simulink library "Source_Lib"  (R2020b)
settings: Solver=VariableStepAuto  StartTime=0.0  StopTime=10.0  RelTol=1e-3
values from neighbouring files (symbols this model uses):
  fb = fn    [Init_Base_SM.m]
  Ib2 = Sb / (3*Vb2)    [Init_Base_SM.m]
undefined symbols (not defined in the file or in its folder): Cmu0, delta0, GOV1_K2, ia0, ib0, ic0, pha0, phb0, phc0, Theta0_deg, Time_Step, V0_pu, Vfu0
libraries: powerlib x41, Control_Lib x14, spsPower3phInstantaneousLib x3, spsSynchronousMachinepuFundamentalLib x2
(part 1 of 2)
settings Model: Creator=abruyere  LastModifiedBy=Frederic_Colas
settings DebuggingCC: ArithmeticOperatorsInVariantConditions=warning
settings SFSimCC: CustomCodeUndefinedFunction=UseInterfaceOnly

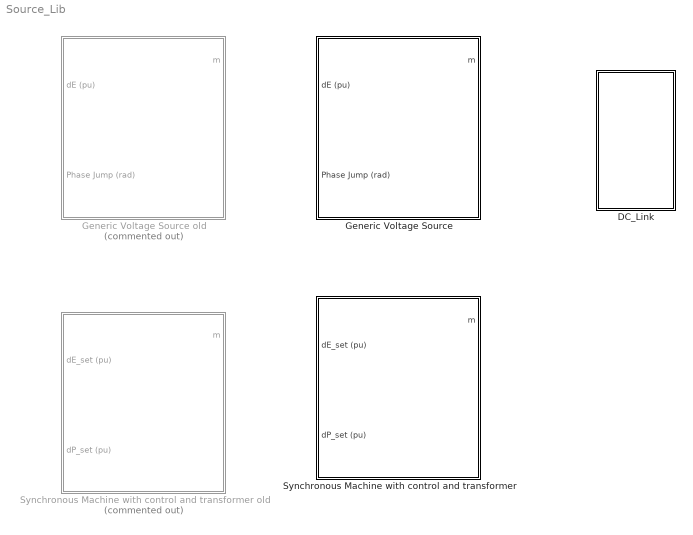
== system Source_Lib ==
  DC_Link : Subsystem  mask{Udc=640e3, Pb=1e6, H_DC=30}
      mask prompts: Udc "Nominal Voltage (V)"; Pb "Nominal Power (W)"; H_DC "DC inertia (ms)"
      mask init:
      | if (H_DC == 0)
      |     set_param([gcb '/C_1'],'Commented','on');
      |     set_param([gcb '/C_2'],'Commented','on');
      |     set_param([gcb '/Udc_1'],'Commented','on');
      |     set_param([gcb '/Udc_2'],'Commented','on');
      | elseif (H_DC == inf)
      |     set_param([gcb '/C_1'],'Commented','on');
      |     set_param([gcb '/C_2'],'Commented','on');
      |     set_param([gcb '/Udc_1'],'Commented','off');
      |     set_param([gcb '/Udc_2'],'Commented','off');
      | else
      |    C_DC = H_DC/1000*Pb/(1/2*Udc^2);
      |    set_param([gcb '/C_1'],'Commented','off','Capacitance',num2str(C_DC*2));
      |    set_param([gcb '/C_2'],'Commented','off','Capacitance',num2str(C_DC*2));
      |    set_param([gcb '/Udc_1'],'Commented','on');
      |    set_param([gcb '/Udc_2'],'Commented','on');
      | end
  Generic Voltage Source : Subsystem  mask(GenericVoltageSource){SourceNature_str=INFINITE, fn=50, Sn=1e9, Un=400e3, H_s=5, DroopOnOff=on, R_percent=4, TN=1, TD=2, Time_Step=50e-6, LFpopup=Swing, P0=0, Q0=0, V0=1, Theta0=0}
      mask prompts: SourceNature_str "Nature of the voltage source"; fn "Nominal frequency fn [Hz]"; Sn "Nominal apparent power Sn [VA]"; Un "Nominal voltage Un [V RMS Ph2Ph]"; H_s "Inertia H [s]"; DroopOnOff "Frequency DROOP activation"; R_percent "Droop gain Kp [%]"; TN "Network time constant Lead [s]"; TD "Network time constant Lag [s]"; Time_Step "Output Delay (s)"; P0 "Active power P0 (pu)"; Q0 "Reactive power Q0 (pu)"; V0 "Initial Voltage (pu)"; Theta0 "Initial angle (°)"
      mask init:
      | % Update Name of LF bus for internal purpose
      | NameStr = [get_param(gcb,'Name')];% '_LF'];
      | set_param([gcb '/Load Flow Bus'],'ID',NameStr);  
      | 
      | % Base specification
      | fb = fn;                % [Hz] base frequency
      | Sb = Sn;                % [VA] base power
      | Ub = Un;                % [V] base ph2ph voltage
      | Vb = Un/sqrt(3);        % [V] base ph2N voltage
      | Ib = Sb/(3*Vb);         % [A] base current
      | Zb = Vb*Ib;             % [Ohm] base impedance
      | 
      | % Set the frequency droop gain
      | R = R_percent / 100;
      | 
      | %Initialize correctly the LoadFlow bus parameters connected to PCC
      |     VLF = V0;
      |     ThetaLF = Theta0;
      |     if (LFpopup == 'PQ')
      |         VLF = 1;
      |         ThetaLF = 0;
      |     elseif (LFpopup == 'PV')
      |         VLF = V0;
      |         ThetaLF = 0;        
      |     end
      |     set_param([gcb '/Load Flow Bus'],'Vref',num2str(VLF),'Vangle',num2str(ThetaLF));
      | 
      | 
      | % Update mask display:
      | % mo = get_param(gcb,'MaskObject');
      | % Generate string to display LF results on Mask
      |     mo = get_param(gcb,'MaskObject');
      |     mo.getDialogControl('LF_pcc_str').Prompt = ['V0 = ', num2str(V0),' pu, Angle = ', num2str(Theta0),'°'];
      |     mo.getDialogControl('LF_pcc_Power_str').Prompt = ['P0 = ', num2str(P0),' pu, Q0 = ', num2str(Q0),' pu'];
      mask TypeOptions SourceNature_str: INFINITE | INERTIAL
      mask Callback SourceNature_str:
      | % Get the mask parameter values. This is a cell
      | %   array of character vectors.
      | maskStr = get_param(gcb,'SourceNature_str');
      | p=Simulink.Mask.get(gcb);
      | 
      | % The pop-up menu is the first mask parameter.
      | %   Check the value selected in the pop-up
      | if strcmp(maskStr,'INFINITE')
      |     p.getDialogControl('Inertial').Visible='off';
      |    %p.getParameter('H_s').Visible='off';
      |    %p.getParameter('DroopOnOff').Visible='off';
      |    %DroopOnOff = 'off';
      |    %p.getParameter('R_percent').Visible='off';
      |    %p.getParameter('TN').Visible='off';
      |    %p.getParameter('TD').Visible='off';
      |    set_param([gcb '/SourceNature'],'Value','1')
      | else
      |    %p.getParameter('H_s').Visible='on';
      |    %p.getParameter('DroopOnOff').Visible='on';
      |    %DroopOnOff = 'on';
      |    %p.getParameter('R_percent').Visible='on';
      |    %p.getParameter('TN').Visible='on';
      |    %p.getParameter('TD').Visible='on';
      |    p.getDialogControl('Inertial').Visible='on';
      |    set_param([gcb '/SourceNature'],'Value','2')
      | end
      mask Callback DroopOnOff:
      | % Get the mask parameter values. This is a cell
      | %   array of character vectors.
      | maskStr = get_param(gcb,'DroopOnOff');
      | p=Simulink.Mask.get(gcb);
      | 
      | if strcmp(maskStr,'on'),
      |     p.getParameter('R_percent').Enabled='on';
      | else
      |     p.getParameter('R_percent').Enabled='off';
      | end
      mask TypeOptions LFpopup: Swing | PQ | PV
      mask Callback LFpopup:
      | % Get the mask parameter values. This is a cell
      | %   array of character vectors.
      | maskStr = get_param(gcb,'LFpopup');
      | p=Simulink.Mask.get(gcb);
      | 
      | % The pop-up menu is the first mask parameter.
      | %   Check the value selected in the pop-up
      | if strcmp(maskStr,'Swing'),
      | 
      |     % Set the visibility of both parameters on when
      |     %   User-defined is selected in the pop-up.
      |     p.getParameter('P0').Visible='off';
      |     p.getParameter('Q0').Visible='off';
      |     p.getParameter('V0').Visible='on';
      |     p.getParameter('Theta0').Visible='on';
      |     set_param([gcb '/Source_For_LF'],'BusType','swing');
      | 
      | elseif strcmp(maskStr,'PQ'),
      | 
      |     % Set the visibility of both parameters on when
      |     %   User-defined is selected in the pop-up.
      |     p.getParameter('P0').Visible='on';
      |     p.getParameter('Q0').Visible='on';
      |     p.getParameter('V0').Visible='off';
      |     p.getParameter('Theta0').Visible='off';
      |     set_param([gcb '/Source_For_LF'],'BusType','PQ');
      | 
      |     % Turn off the visibility of the Value field
      |     %   when User-defined is not selected.
      | else
      | 
      |     % Set the visibility of both parameters on when
      |     %   User-defined is selected in the pop-up.
      |     p.getParameter('P0').Visible='on';
      |     p.getParameter('Q0').Visible='off';
      |     p.getParameter('V0').Visible='on';
      |     p.getParameter('Theta0').Visible='off';
      |     set_param([gcb '/Source_For_LF'],'BusType','PV');
      | 
      | end
      mask DialogControl Container8 Prompt: Nominal Value
      mask DialogControl Inertial Prompt: Inertial source parameters
      mask DialogControl LF_Param Prompt: Loadflow
      mask DialogControl Control1 Prompt: Initial Operating Point
      mask DialogControl Container6 Prompt: PCC
      mask DialogControl LF_pcc_str Prompt: V0 = 1 pu, Angle = 0°
      mask DialogControl LF_pcc_Power_str Prompt: P0 = 0 pu, Q0 = 0 pu
      mask DialogControl Control4 Prompt: Update Loadflow
      mask DialogControl Control4 Callback: LoadFlow_VSC
      mask Display:
      | if (SourceNature_str == 1)
      |     image(imread('infinite.png'));
      |     color('blue')
      |     text(0.3,0.10,'Infinite bus')
      | else
      |     image(imread('inertia.png'));
      |     color('blue')
      |     text(0.3,0.10,'Inertia Emulation')
      | end
      | 
      | port_label('input',1,'\DeltaE (pu)','texmode','on');
      | port_label('input',2,'\Delta\theta (rad)','texmode','on');
      | port_label('output',1,'m');
      | port_label('rconn',1,'A');
      | port_label('rconn',2,'B');
      | port_label('rconn',3,'C');
  Generic Voltage Source old : Subsystem  Commented=on  mask(GenericVoltageSource){SourceNature_str=INFINITE, fn=50, Sn=1e9, Un=400e3, Time_Step=Time_Step, H_s=5, DroopOnOff=on, R_percent=4, TN=1, TD=2, LFpopup=Swing, P0=-491545376.7896, Q0=82825649.5509, V0=1, Theta0=0}
      mask prompts: SourceNature_str "Nature of the voltage source"; fn "Nominal frequency fn [Hz]"; Sn "Nominal apparent power Sn [VA]"; Un "Nominal voltage Un [V RMS Ph2Ph]"; Time_Step "Sample Time (s)"; H_s "Inertia H [s]"; DroopOnOff "Frequency DROOP activation"; R_percent "Droop gain Kp [%]"; TN "Network time constant Lead [s]"; TD "Network time constant Lag [s]"; P0 "Active power P0 (pu)"; Q0 "Reactive power Q0 (pu)"; V0 "Initial Voltage (pu)"; Theta0 "Initial angle (°)"
      mask init:
      | % Update Name of LF bus for internal purpose
      | NameStr = [get_param(gcb,'Name')];% '_LF'];
      | set_param([gcb '/Load Flow Bus'],'ID',NameStr);  
      | 
      | % Base specification
      | fb = fn;                % [Hz] base frequency
      | Sb = Sn;                % [VA] base power
      | Ub = Un;                % [V] base ph2ph voltage
      | Vb = Un/sqrt(3);        % [V] base ph2N voltage
      | Ib = Sb/(3*Vb);         % [A] base current
      | Zb = Vb*Ib;             % [Ohm] base impedance
      | 
      | % Set the frequency droop gain
      | R = R_percent / 100;
      | 
      | %Initialize correctly the LoadFlow bus parameters connected to PCC
      |     VLF = V0_pu;
      |     ThetaLF = Theta0_deg;
      |     if (LFpopup == 'PQ')
      |         VLF = 1;
      |         ThetaLF = 0;
      |     elseif (LFpopup == 'PV')
      |         VLF = V0_pu;
      |         ThetaLF = 0;        
      |     end
      |     set_param([gcb '/Load Flow Bus'],'Vref',num2str(VLF),'Vangle',num2str(ThetaLF));
      | 
      | 
      | % Update mask display:
      | % mo = get_param(gcb,'MaskObject');
      mask TypeOptions SourceNature_str: INFINITE | INERTIAL
      mask Callback SourceNature_str:
      | % Get the mask parameter values. This is a cell
      | %   array of character vectors.
      | maskStr = get_param(gcb,'SourceNature_str');
      | p=Simulink.Mask.get(gcb);
      | 
      | % The pop-up menu is the first mask parameter.
      | %   Check the value selected in the pop-up
      | if strcmp(maskStr,'INFINITE')
      |     p.getDialogControl('Inertial').Visible='off';
      |    %p.getParameter('H_s').Visible='off';
      |    %p.getParameter('DroopOnOff').Visible='off';
      |    %DroopOnOff = 'off';
      |    %p.getParameter('R_percent').Visible='off';
      |    %p.getParameter('TN').Visible='off';
      |    %p.getParameter('TD').Visible='off';
      |    set_param([gcb '/SourceNature'],'Value','1')
      | else
      |    %p.getParameter('H_s').Visible='on';
      |    %p.getParameter('DroopOnOff').Visible='on';
      |    %DroopOnOff = 'on';
      |    %p.getParameter('R_percent').Visible='on';
      |    %p.getParameter('TN').Visible='on';
      |    %p.getParameter('TD').Visible='on';
      |    p.getDialogControl('Inertial').Visible='on';
      |    set_param([gcb '/SourceNature'],'Value','2')
      | end
      mask Callback DroopOnOff:
      | % Get the mask parameter values. This is a cell
      | %   array of character vectors.
      | maskStr = get_param(gcb,'DroopOnOff');
      | p=Simulink.Mask.get(gcb);
      | 
      | if strcmp(maskStr,'on'),
      |     p.getParameter('R_percent').Enabled='on';
      | else
      |     p.getParameter('R_percent').Enabled='off';
      | end
      mask TypeOptions LFpopup: Swing | PQ | PV
      mask Callback LFpopup:
      | % Get the mask parameter values. This is a cell
      | %   array of character vectors.
      | maskStr = get_param(gcb,'LFpopup');
      | p=Simulink.Mask.get(gcb);
      | 
      | % The pop-up menu is the first mask parameter.
      | %   Check the value selected in the pop-up
      | if strcmp(maskStr,'Swing'),
      | 
      |     % Set the visibility of both parameters on when
      |     %   User-defined is selected in the pop-up.
      |     p.getParameter('P0').Visible='off';
      |     p.getParameter('Q0').Visible='off';
      |     p.getParameter('V0').Visible='on';
      |     p.getParameter('Theta0').Visible='on';
      |     set_param([gcb '/Source_For_LF'],'BusType','swing');
      | 
      | elseif strcmp(maskStr,'PQ'),
      | 
      |     % Set the visibility of both parameters on when
      |     %   User-defined is selected in the pop-up.
      |     p.getParameter('P0').Visible='on';
      |     p.getParameter('Q0').Visible='on';
      |     p.getParameter('V0').Visible='off';
      |     p.getParameter('Theta0').Visible='off';
      |     set_param([gcb '/Source_For_LF'],'BusType','PQ');
      | 
      |     % Turn off the visibility of the Value field
      |     %   when User-defined is not selected.
      | else
      | 
      |     % Set the visibility of both parameters on when
      |     %   User-defined is selected in the pop-up.
      |     p.getParameter('P0').Visible='on';
      |     p.getParameter('Q0').Visible='off';
      |     p.getParameter('V0').Visible='on';
      |     p.getParameter('Theta0').Visible='off';
      |     set_param([gcb '/Source_For_LF'],'BusType','PV');
      | 
      | end
      mask DialogControl Container8 Prompt: Nominal Value
      mask DialogControl Inertial Prompt: Inertial source parameters
      mask DialogControl LF_Param Prompt: Loadflow
      mask Display:
      | if (SourceNature_str == 1)
      |     image(imread('infinite.png'));
      |     color('blue')
      |     text(0.3,0.10,'Infinite bus')
      | else
      |     image(imread('inertia.png'));
      |     color('blue')
      |     text(0.3,0.10,'Inertia Emulation')
      | end
      | 
      | port_label('input',1,'\DeltaE (pu)','texmode','on');
      | port_label('input',2,'\Delta\theta (rad)','texmode','on');
      | port_label('output',1,'m');
      | port_label('rconn',1,'A');
      | port_label('rconn',2,'B');
      | port_label('rconn',3,'C');
  Synchronous Machine with control and transformer : Subsystem  mask(SM){Sn=900e6, Pn=900e6, fn=50, SM_Unom=20e3, Paux=0.01, SM_Rs=0.0025, SM_Ll=0.2, SM_Lmd=1.6, SM_Lmq=1.5, SM_Rf=0.006, SM_Llfd=0.1067, SM_Rkd=0.0177, SM_Llkd=0.1, SM_Rkq1=0.013, SM_Llkq1=0.4565, SM_Rkq2=0.0217, SM_Llkq2=0.0583, SM_H=6.5, SM_F=0, SM_p=1, Un1=20e3, Un2=400e3, Rt_pu=0, Lt_pu=0.15, Lm_pu=500, Rm_pu=500, GOV_Kpf=-25, GOV_tau1=0.1, GOV_tau3=0.2, GOV_tau4=0.05, GOV_K2=0.7, GOV_tau5=7, GOV_K3=0.4, GOV_tau6=0.4, ST1_Ka=200, ST1_taur=0.01, OP_Vfu=0, PSS_K=20, PSS_tau1=0.05, PSS_tau2=0.02, PSS_tau3=3, PSS_tau4=5.4, PSS_tau5=0.05, PSS_tau6=0.01, LFpopup=PV, P0=0.9, Q0=-0.064025, V0=1, Theta0=3.6743}
      mask prompts: Sn "Nominal apparent power (VA)"; Pn "Nominal active power (W)"; fn "Frequency (Hz)"; SM_Unom "Line-to-line voltage (Vrms)"; Paux "Auxilary charge  (p.u)"; SM_Rs "Stator resistance : Rs(pu)"; SM_Ll "Stator leakage inductance : Ll(pu)"; SM_Lmd "Magnetic inductance in d-axis  : Lmd(pu)"; SM_Lmq "Magnetic inductance in q-axis  : Lmq(pu)"; SM_Rf "Field resistance : Rf(pu)"; SM_Llfd "Field leakage inductance  : Llfd(pu)"; SM_Rkd "d-axis damper resistance : Rkd(pu)"; SM_Llkd "d-axis damper leakage inductance : Llkd(pu)"; SM_Rkq1 "1st q-axis damper resistance:  Rkq1(pu)"; SM_Llkq1 "1st q-axis damper leakage inductance : Lkq1(pu)"; SM_Rkq2 "2nd  q-axis damper resistance :  Rkq2(pu)"; SM_Llkq2 "2nd q-axis damper leakage inductance :  Llkq2(pu)"; SM_H "Inertia coefficient : H(s)"; SM_F "Friction  factor : F(pu)"; SM_p "Poles pairs : p()"; Un1 "Primary line-to-line voltage (Vrms)"; Un2 "Secondary line-to-line voltage (Vrms)"; Rt_pu "Resistance : R(pu)"; Lt_pu "Leakage inductance : L(pu)"; Lm_pu "Magnetization resistance : Rm(pu)"; Rm_pu "Magnetization resistance : Lm(pu)"; GOV_Kpf "Power frecuency characteristic : Kpf"; GOV_tau1 "Lag time constant : tau1(s)"; GOV_tau3 "Lag time constant : tau3(s)"; GOV_tau4 "Steam flow time constant : tau4(s)"; GOV_K2 "Intermediary Pressure Reheater power fraction : K2"; GOV_tau5 "Intermediary Pressure Reheater time constant : tau5(s)"; GOV_K3 "Low Pressure Reheater power fraction : K3"; GOV_tau6 "Intermediary Pressure Reheater time constant : tau6(s)"; ST1_Ka "Main regulator gain : Ka"; ST1_taur "Filter time constant : taur(s)"; PSS_K "Gain"; PSS_tau1 "tau1"; PSS_tau2 "tau2"; PSS_tau3 "tau3"; PSS_tau4 "tau4"; PSS_tau5 "tau5"; PSS_tau6 "tau6"; P0 "Initial Active Power (pu)"; Q0 "Initial Reactive Power (pu)"; V0 "Initial Voltage (pu)"; Theta0 "Initial Angle (°)"
      mask init:
      | Init_Base_SM;
      | Init_LF_SM;
      | Init_SM;
      mask TypeOptions LFpopup: Swing | PQ | PV
      mask Callback LFpopup:
      | % Get the mask parameter values. This is a cell
      | %   array of character vectors.
      | maskStr = get_param(gcb,'LFpopup');
      | p=Simulink.Mask.get(gcb);
      | 
      | % The pop-up menu is the first mask parameter.
      | %   Check the value selected in the pop-up
      | if strcmp(maskStr,'Swing'),
      | 
      |     % Set the visibility of both parameters on when
      |     %   User-defined is selected in the pop-up.
      |     p.getParameter('P0').Visible='off';
      |     p.getParameter('Q0').Visible='off';
      |     p.getParameter('V0').Visible='on';
      |     p.getParameter('Theta0').Visible='on';
      |     set_param([gcb '/Source_For_LF'],'BusType','swing');
      | 
      | elseif strcmp(maskStr,'PQ'),
      | 
      |     % Set the visibility of both parameters on when
      |     %   User-defined is selected in the pop-up.
      |     p.getParameter('P0').Visible='on';
      |     p.getParameter('Q0').Visible='on';
      |     p.getParameter('V0').Visible='off';
      |     p.getParameter('Theta0').Visible='off';
      |     set_param([gcb '/Source_For_LF'],'BusType','PQ');
      | 
      |     % Turn off the visibility of the Value field
      |     %   when User-defined is not selected.
      | else
      | 
      |     % Set the visibility of both parameters on when
      |     %   User-defined is selected in the pop-up.
      |     p.getParameter('P0').Visible='on';
      |     p.getParameter('Q0').Visible='off';
      |     p.getParameter('V0').Visible='on';
      |     p.getParameter('Theta0').Visible='off';
      |     set_param([gcb '/Source_For_LF'],'BusType','PV');
      | 
      | end
      mask DialogControl SM_param Prompt: SM
      mask DialogControl Container16 Prompt: On the synchronous machine
      mask DialogControl Control2 Prompt: Parameters for a Round rotor machine with Pm as mechanical inputs
      mask DialogControl SM_nomV Prompt: Nominal Values
      mask DialogControl SM_stator Prompt: Stator
      mask DialogControl SM_field Prompt: Field
      mask DialogControl SM_dampers Prompt: Dampers
      mask DialogControl SM_mech Prompt: Mechanical
      mask DialogControl Container15 Prompt: TR
      mask DialogControl Container14 Prompt: On the transformer.
      mask DialogControl Control_TR Prompt: Yg-Yg Three sinle phase transformers. Parameters gather on the secondary side.
      mask DialogControl GOV_param Prompt: GOV
      mask DialogControl Container18 Prompt: On the governor
      mask DialogControl Control5 Prompt: IEESGO
      mask DialogControl Container20 Prompt: Parameters
      mask DialogControl ST1_param Prompt: ST1
      mask DialogControl Container22 Prompt: On the excitation system
      mask DialogControl Control6 Prompt: Simplified ST1A from IEEE stantard
      mask DialogControl Exc_param Prompt: Parameters
      mask DialogControl PSS_param Prompt: PSS
      mask DialogControl Container11 Prompt: Loadflow
      mask DialogControl Control4 Prompt: Initial Operating Point
      mask DialogControl Container24 Prompt: VSC side
      mask DialogControl LF_vsc_str Prompt: V0 = 0.99971 pu, Angle = 15.1187°
      mask DialogControl Container25 Prompt: PCC
      mask DialogControl LF_pcc_str Prompt: V0 = 1 pu, Angle = 3.6743°
      mask DialogControl LF_pcc_Power_str Prompt: P0 = 0.9 pu, Q0 = -0.064025 pu
      mask DialogControl UpdateLoadflow Prompt: Update Loadflow
      mask DialogControl UpdateLoadflow Callback: LoadFlow_VSC
      mask Display:
      | image(imread('inertia.png'));
      | color('blue');
      | text(0.3,0.10,'SM with control \n+ transfomer');
      | 
      | port_label('input',1,'\DeltaE (pu)','texmode','on');
      | port_label('input',2,'\Delta\theta (rad)','texmode','on');
      | port_label('output',1,'m');
      | port_label('rconn',1,'A');
      | port_label('rconn',2,'B');
      | port_label('rconn',3,'C');
  Synchronous Machine with control and transformer old : Subsystem  Commented=on  mask(SM){Sn=900e6, Pn=900e6, fn=50, SM_Unom=20e3, Paux=0.01, SM_Rs=0.0025, SM_Ll=0.2, SM_Lmd=1.6, SM_Lmq=1.5, SM_Rf=0.006, SM_Llfd=0.1067, SM_Rkd=0.0177, SM_Llkd=0.1, SM_Rkq1=0.013, SM_Llkq1=0.4565, SM_Rkq2=0.0217, SM_Llkq2=0.0583, SM_H=6.5, SM_F=0, SM_p=1, Un1=20e3, Un2=230e3, Rt_pu=0, Lt_pu=0.15, Lm_pu=500, Rm_pu=500, GOV_Kpf=-25, GOV_tau1=0.1, GOV_tau3=0.2, GOV_tau4=0.05, GOV_K2=0.7, GOV_tau5=7, GOV_K3=0.4, GOV_tau6=0.4, ST1_Ka=200, ST1_taur=0.01, OP_Vfu=0, PSS_K=20, PSS_tau1=0.05, PSS_tau2=0.02, PSS_tau3=3, PSS_tau4=5.4, PSS_tau5=0.05, PSS_tau6=0.01, LFpopup=PV, P0=0.7, Q0=-0.047626, V0=1, Theta0=3.6366}
      mask prompts: Sn "Nominal apparent power (VA)"; Pn "Nominal active power (W)"; fn "Frequency (Hz)"; SM_Unom "Line-to-line voltage (Vrms)"; Paux "Auxilary charge  (p.u)"; SM_Rs "Stator resistance : Rs(pu)"; SM_Ll "Stator leakage inductance : Ll(pu)"; SM_Lmd "Magnetic inductance in d-axis  : Lmd(pu)"; SM_Lmq "Magnetic inductance in q-axis  : Lmq(pu)"; SM_Rf "Field resistance : Rf(pu)"; SM_Llfd "Field leakage inductance  : Llfd(pu)"; SM_Rkd "d-axis damper resistance : Rkd(pu)"; SM_Llkd "d-axis damper leakage inductance : Llkd(pu)"; SM_Rkq1 "1st q-axis damper resistance:  Rkq1(pu)"; SM_Llkq1 "1st q-axis damper leakage inductance : Lkq1(pu)"; SM_Rkq2 "2nd  q-axis damper resistance :  Rkq2(pu)"; SM_Llkq2 "2nd q-axis damper leakage inductance :  Llkq2(pu)"; SM_H "Inertia coefficient : H(s)"; SM_F "Friction  factor : F(pu)"; SM_p "Poles pairs : p()"; Un1 "Primary line-to-line voltage (Vrms)"; Un2 "Secondary line-to-line voltage (Vrms)"; Rt_pu "Resistance : R(pu)"; Lt_pu "Leakage inductance : L(pu)"; Lm_pu "Magnetization resistance : Rm(pu)"; Rm_pu "Magnetization resistance : Lm(pu)"; GOV_Kpf "Power frecuency characteristic : Kpf"; GOV_tau1 "Lag time constant : tau1(s)"; GOV_tau3 "Lag time constant : tau3(s)"; GOV_tau4 "Steam flow time constant : tau4(s)"; GOV_K2 "Intermediary Pressure Reheater power fraction : K2"; GOV_tau5 "Intermediary Pressure Reheater time constant : tau5(s)"; GOV_K3 "Low Pressure Reheater power fraction : K3"; GOV_tau6 "Intermediary Pressure Reheater time constant : tau6(s)"; ST1_Ka "Main regulator gain : Ka"; ST1_taur "Filter time constant : taur(s)"; PSS_K "Gain"; PSS_tau1 "tau1"; PSS_tau2 "tau2"; PSS_tau3 "tau3"; PSS_tau4 "tau4"; PSS_tau5 "tau5"; PSS_tau6 "tau6"; P0 "Initial Active Power (pu)"; Q0 "Initial Reactive Power (pu)"; V0 "Initial Voltage (pu)"; Theta0 "Initial Angle (°)"
      mask init:
      | Init_Base_SM;
      | Init_LF_SM;
      | Init_SM;
      mask TypeOptions LFpopup: Swing | PQ | PV
      mask Callback LFpopup:
      | % Get the mask parameter values. This is a cell
      | %   array of character vectors.
      | maskStr = get_param(gcb,'LFpopup');
      | p=Simulink.Mask.get(gcb);
      | 
      | % The pop-up menu is the first mask parameter.
      | %   Check the value selected in the pop-up
      | if strcmp(maskStr,'Swing'),
      | 
      |     % Set the visibility of both parameters on when
      |     %   User-defined is selected in the pop-up.
      |     p.getParameter('P0').Visible='off';
      |     p.getParameter('Q0').Visible='off';
      |     p.getParameter('V0').Visible='on';
      |     p.getParameter('Theta0').Visible='on';
      |     set_param([gcb '/Source_For_LF'],'BusType','swing');
      | 
      | elseif strcmp(maskStr,'PQ'),
      | 
      |     % Set the visibility of both parameters on when
      |     %   User-defined is selected in the pop-up.
      |     p.getParameter('P0').Visible='on';
      |     p.getParameter('Q0').Visible='on';
      |     p.getParameter('V0').Visible='off';
      |     p.getParameter('Theta0').Visible='off';
      |     set_param([gcb '/Source_For_LF'],'BusType','PQ');
      | 
      |     % Turn off the visibility of the Value field
      |     %   when User-defined is not selected.
      | else
      | 
      |     % Set the visibility of both parameters on when
      |     %   User-defined is selected in the pop-up.
      |     p.getParameter('P0').Visible='on';
      |     p.getParameter('Q0').Visible='off';
      |     p.getParameter('V0').Visible='on';
      |     p.getParameter('Theta0').Visible='off';
      |     set_param([gcb '/Source_For_LF'],'BusType','PV');
      | 
      | end
      mask DialogControl SM_param Prompt: SM
      mask DialogControl Container16 Prompt: On the synchronous machine
      mask DialogControl Control2 Prompt: Parameters for a Round rotor machine with Pm as mechanical inputs
      mask DialogControl SM_nomV Prompt: Nominal Values
      mask DialogControl SM_stator Prompt: Stator
      mask DialogControl SM_field Prompt: Field
      mask DialogControl SM_dampers Prompt: Dampers
      mask DialogControl SM_mech Prompt: Mechanical
      mask DialogControl Container15 Prompt: TR
      mask DialogControl Container14 Prompt: On the transformer.
      mask DialogControl Control_TR Prompt: Yg-Yg Three sinle phase transformers. Parameters gather on the secondary side.
      mask DialogControl GOV_param Prompt: GOV
      mask DialogControl Container18 Prompt: On the governor
      mask DialogControl Control5 Prompt: IEESGO
      mask DialogControl Container20 Prompt: Parameters
      mask DialogControl ST1_param Prompt: ST1
      mask DialogControl Container22 Prompt: On the excitation system
      mask DialogControl Control6 Prompt: Simplified ST1A from IEEE stantard
      mask DialogControl Exc_param Prompt: Parameters
      mask DialogControl PSS_param Prompt: PSS
      mask DialogControl Container11 Prompt: Loadflow
      mask DialogControl Control4 Prompt: Initial Operating Point
      mask DialogControl Container24 Prompt: VSC side
      mask DialogControl LF_vsc_str Prompt: V0 = 0.99855 pu, Angle = 13.3182°
      mask DialogControl Container25 Prompt: PCC
      mask DialogControl LF_pcc_str Prompt: V0 = 1 pu, Angle = 3.6366°
      mask DialogControl LF_pcc_Power_str Prompt: P0 = 0.7 pu, Q0 = -0.047626 pu
      mask DialogControl UpdateLoadflow Prompt: Update Loadflow
      mask DialogControl UpdateLoadflow Callback: LoadFlow_VSC
      mask Display:
      | image(imread('inertia.png'));
      | color('blue');
      | text(0.3,0.10,'SM with control \n+ transfomer');
      | 
      | port_label('input',1,'\DeltaE (pu)','texmode','on');
      | port_label('input',2,'\Delta\theta (rad)','texmode','on');
      | port_label('output',1,'m');
      | port_label('rconn',1,'A');
      | port_label('rconn',2,'B');
      | port_label('rconn',3,'C');

== system Source_Lib/DC_Link ==
  C_1 : powerlib/Elements/Series RLC Branch  LConnTagsString=__new0  RConnTagsString=__new0  BranchType=C  Resistance=1  Inductance=1e-3  SetiL0=off  InitialCurrent=0  Capacitance=2.9297e-07  Setx0=on  InitialVoltage=Udc/2  Measurements=None
  C_2 : powerlib/Elements/Series RLC Branch  LConnTagsString=__new0  RConnTagsString=__new0  BranchType=C  Resistance=1  Inductance=1e-3  SetiL0=off  InitialCurrent=0  Capacitance=2.9297e-07  Setx0=on  InitialVoltage=Udc/2  Measurements=None
  Udc_1 : powerlib/Electrical Sources/DC Voltage Source  Commented=on  Amplitude=Udc/2  Measurements=None
  Udc_2 : powerlib/Electrical Sources/DC Voltage Source  Commented=on  Amplitude=Udc/2  Measurements=None
  + : PMIOPort  Side=Right
  0 : PMIOPort  Port=2  Side=Right
  - : PMIOPort  Port=3  Side=Right
  connections:
  Udc_2/LConn1 -- C_2/RConn1 -- -/RConn1
  Udc_1/RConn1 -- C_1/LConn1 -- +/RConn1
  0/RConn1 -- C_2/LConn1 -- C_1/RConn1 -- Udc_2/RConn1 -- Udc_1/LConn1

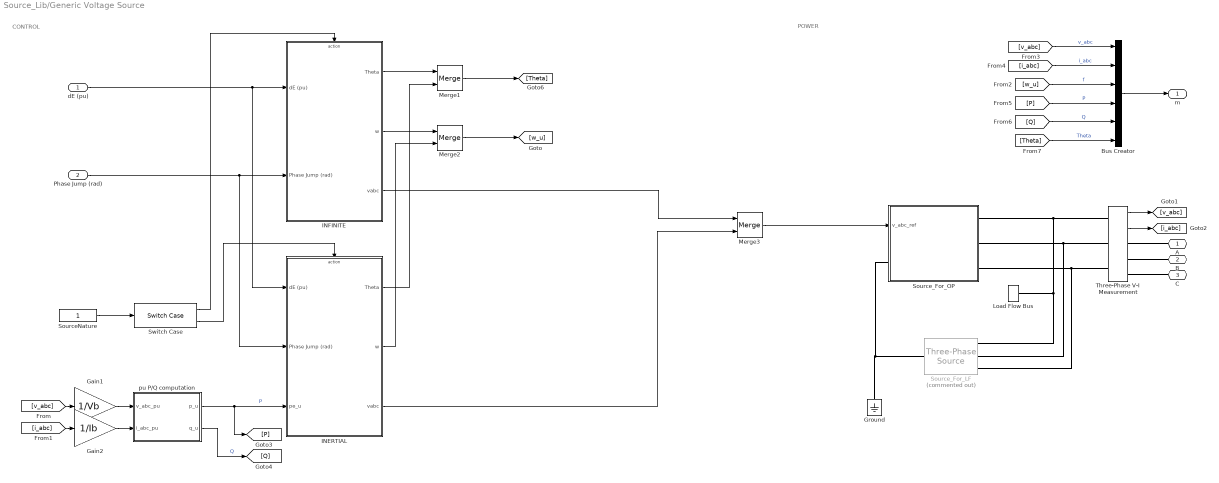
== system Source_Lib/Generic Voltage Source ==
  note: POWER
  note: CONTROL
  dE (pu) : Inport
  Phase Jump (rad) : Inport  Port=2
  " pu P/Q computation" : Subsystem  DialogController=POWERSYS.PowerSysDialog
  Bus Creator : BusCreator  Inputs=6
  Gain1 : Gain  Gain=1/Vb
  Gain2 : Gain  Gain=1/Ib
  Ground : powerlib/Elements/Ground  LConnTagsString=a
  INERTIAL : Subsystem
  INFINITE : Subsystem
  Load Flow Bus : powerlib/Measurements/Load Flow Bus  LConnTagsString=a  Phases=single  Connectors=on one side  ID=Generic Voltage Source  Vbase=Un  Vref=1  Vangle=0  VLF=1  VLFb=1  VLFc=1  angleLF=0  angleLFb=0  angleLFc=0
  Merge1 : Merge
  Merge2 : Merge
  Merge3 : Merge
  SourceNature : Constant
  Source_For_LF : powerlib/Electrical Sources/Three-Phase Source  Commented=on  InternalConnection=Yn  VoltagePhases=off  Voltage=(400000)*1  PhaseAngle=0  Voltage_phases=[25e3 25e3 25e3]/sqrt(3)  PhaseAngles_phases=[0 -120 +120]  Frequency=fb  NonIdealSource=off  SpecifyImpedance=off  Resistance=0  Inductance=0  ShortCircuitLevel=100e6  BaseVoltage=Un  XRratio=7  BusType=swing  Pref=P0*Sb  Qref=Q0*Sb  Prefabc=[10e3, 10e3, 10e3]  Qrefabc=[0, 0, 0]  Qmin=-inf  Qmax=inf
  Source_For_OP : Subsystem
  Switch Case : SwitchCase  CaseConditions={1, 2}  ShowDefaultCase=off
  Three-Phase V-I Measurement : powerlib/Measurements/Three-Phase V-I Measurement  VoltageMeasurement=phase-to-ground  SetLabelV=off  LabelV=v_abc  Vpu=off  VpuLL=off  CurrentMeasurement=yes  SetLabelI=off  LabelI=i_abc  Ipu=off  Pbase=100e6  Vbase=500e3  OutputType=Complex  PhasorSimulation=off  PSBequivalent=0
  A : PMIOPort  Side=Right
  B : PMIOPort  Port=2  Side=Right
  C : PMIOPort  Port=3  Side=Right
  m : Outport  VectorParamsAs1DForOutWhenUnconnected=off
  wires:
  [Q] -> Bus Creator/5  "Q"
  [P] -> Bus Creator/4  "P"
  Three-Phase V-I Measurement/2 -> [i_abc]
  Three-Phase V-I Measurement/1 -> [v_abc]
  Bus Creator/1 -> m/1
  [w_u] -> Bus Creator/3  "f"
  [i_abc] -> Bus Creator/2  "i_abc"
  [v_abc] -> Bus Creator/1  "v_abc"
  " pu P/Q computation"/1(p_u) -> INERTIAL/3(pe_u), [P]  "P"
  " pu P/Q computation"/2(q_u) -> [Q]  "Q"
  Gain2/1 -> " pu P/Q computation"/2(i_abc_pu)
  Gain1/1 -> " pu P/Q computation"/1(v_abc_pu)
  [i_abc] -> Gain2/1
  [v_abc] -> Gain1/1
  Switch Case/2 -> INERTIAL/Action
  Switch Case/1 -> INFINITE/Action
  SourceNature/1 -> Switch Case/1
  [Theta] -> Bus Creator/6  "Theta"
  INFINITE/1(Theta) -> Merge1/1
  Merge1/1 -> [Theta]
  dE (pu)/1 -> INERTIAL/1(dE (pu)), INFINITE/1(dE (pu))
  Phase Jump (rad)/1 -> INERTIAL/2(Phase Jump (rad)), INFINITE/2(Phase Jump (rad))
  INERTIAL/1(Theta) -> Merge1/2
  INFINITE/2(w) -> Merge2/1
  INERTIAL/2(w) -> Merge2/2
  Merge2/1 -> [w_u]
  Merge3/1 -> Source_For_OP/1(v_abc_ref)
  INFINITE/3(vabc) -> Merge3/1
  INERTIAL/3(vabc) -> Merge3/2
  connections:
  Three-Phase V-I Measurement/RConn3 -- C/RConn1
  Three-Phase V-I Measurement/RConn2 -- B/RConn1
  Three-Phase V-I Measurement/RConn1 -- A/RConn1
  Three-Phase V-I Measurement/LConn1 -- Load Flow Bus/LConn1 -- Source_For_LF/RConn1 -- Source_For_OP/RConn1
  Source_For_OP/RConn3 -- Three-Phase V-I Measurement/LConn3 -- Source_For_LF/RConn3
  Source_For_LF/LConn1 -- Ground/LConn1 -- Source_For_OP/LConn1
  Source_For_OP/RConn2 -- Three-Phase V-I Measurement/LConn2 -- Source_For_LF/RConn2

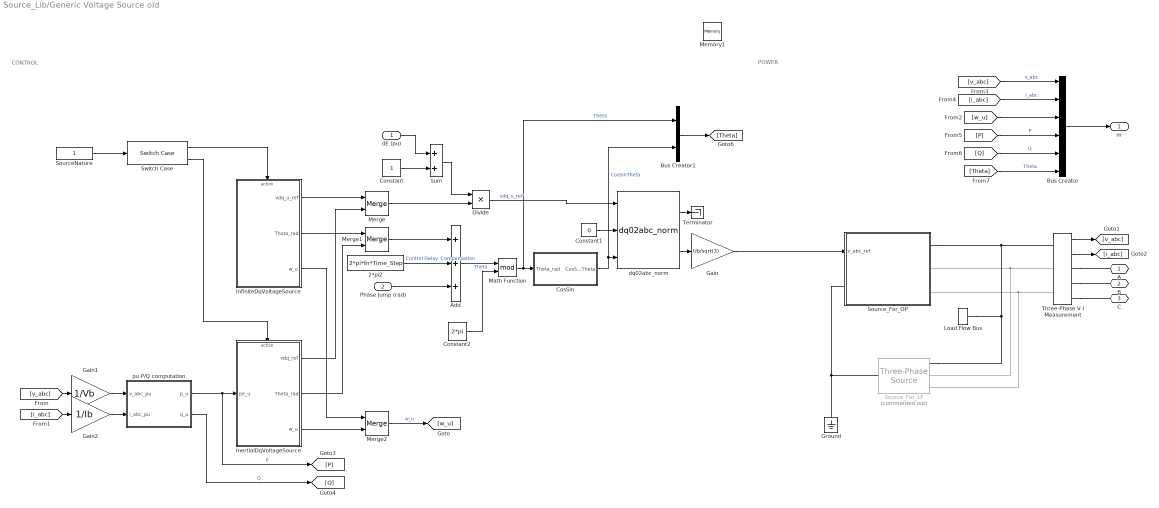
== system Source_Lib/Generic Voltage Source old ==
  note: CONTROL
  note: POWER
  dE (pu) : Inport
  Phase Jump (rad) : Inport  Port=2
  " pu P/Q computation" : Subsystem  DialogController=POWERSYS.PowerSysDialog
  2*pi2 : Constant  Value=2*pi*fn*Time_Step
  Add : Sum  Inputs=+++
  Bus Creator : BusCreator  Inputs=6
  Bus Creator1 : BusCreator  Inputs=2
  Constant : Constant
  Constant1 : Constant  Value=0
  Constant2 : Constant  Value=2*pi
  CosSin : Subsystem
  Divide : Product  Inputs=**
  Gain : Gain  Gain=Ub/sqrt(3)
  Gain1 : Gain  Gain=1/Vb
  Gain2 : Gain  Gain=1/Ib
  Ground : powerlib/Elements/Ground  LConnTagsString=a
  InertialDqVoltageSource : Subsystem  TreatAsAtomicUnit=on
  InfiniteDqVoltageSource : Subsystem  TreatAsAtomicUnit=on
  Load Flow Bus : powerlib/Measurements/Load Flow Bus  LConnTagsString=a  Phases=single  Connectors=on one side  ID=Generic Voltage Source old  Vbase=Un  Vref=1  Vangle=0  VLF=1  VLFb=1  VLFc=1  angleLF=0  angleLFb=0  angleLFc=0
  Math Function : Math  Operator=mod  SaturateOnIntegerOverflow=on
  Memory1 : Memory
  Merge : Merge
  Merge1 : Merge
  Merge2 : Merge
  SourceNature : Constant
  Source_For_LF : powerlib/Electrical Sources/Three-Phase Source  Commented=on  InternalConnection=Yn  VoltagePhases=off  Voltage=(400000)*1  PhaseAngle=0  Voltage_phases=[25e3 25e3 25e3]/sqrt(3)  PhaseAngles_phases=[0 -120 +120]  Frequency=fb  NonIdealSource=off  SpecifyImpedance=off  Resistance=0  Inductance=0  ShortCircuitLevel=100e6  BaseVoltage=Un  XRratio=7  BusType=swing  Pref=P0  Qref=Q0  Prefabc=[10e3, 10e3, 10e3]  Qrefabc=[0, 0, 0]  Qmin=-inf  Qmax=inf
  Source_For_OP : Subsystem
  Sum : Sum
  Switch Case : SwitchCase  CaseConditions={1, 2}  ShowDefaultCase=off
  Terminator : Terminator
  Three-Phase V-I Measurement : powerlib/Measurements/Three-Phase V-I Measurement  VoltageMeasurement=phase-to-ground  SetLabelV=off  LabelV=v_abc  Vpu=off  VpuLL=off  CurrentMeasurement=yes  SetLabelI=off  LabelI=i_abc  Ipu=off  Pbase=100e6  Vbase=500e3  OutputType=Complex  PhasorSimulation=off  PSBequivalent=0
  dq02abc_norm : Control_Lib/dq02abc_norm  referenceAxisMode=Reference axis at 90 degrees behind phase_a  baseUpdateGain=sqrt(3)
      settings: SourceProductName=VSC_Lib
  A : PMIOPort  Side=Right
  B : PMIOPort  Port=2  Side=Right
  C : PMIOPort  Port=3  Side=Right
  m : Outport  VectorParamsAs1DForOutWhenUnconnected=off
  wires:
  Phase Jump (rad)/1 -> Add/3
  [Theta] -> Bus Creator/6  "Theta"
  Bus Creator1/1 -> [Theta]
  dq02abc_norm/2 -> Gain/1
  Constant1/1 -> dq02abc_norm/2
  dq02abc_norm/1 -> Terminator/1
  SourceNature/1 -> Switch Case/1
  Switch Case/1 -> InfiniteDqVoltageSource/Action
  InfiniteDqVoltageSource/1(vdq_u_ref) -> Merge/1
  InertialDqVoltageSource/1(vdq_ref) -> Merge/2
  Merge/1 -> Divide/2
  InfiniteDqVoltageSource/2(Theta_rad) -> Merge1/1
  InertialDqVoltageSource/2(Theta_rad) -> Merge1/2
  Switch Case/2 -> InertialDqVoltageSource/Action
  [v_abc] -> Gain1/1
  [i_abc] -> Gain2/1
  Gain1/1 -> " pu P/Q computation"/1(v_abc_pu)
  Gain2/1 -> " pu P/Q computation"/2(i_abc_pu)
  CosSin/1(CosSinTheta) -> dq02abc_norm/3, Bus Creator1/2  "CosSinTheta"
  " pu P/Q computation"/2(q_u) -> [Q]  "Q"
  " pu P/Q computation"/1(p_u) -> InertialDqVoltageSource/1(pe_u), [P]  "P"
  Gain/1 -> Source_For_OP/1(v_abc_ref)
  Math Function/1 -> Bus Creator1/1, CosSin/1(Theta_rad)  "Theta"
  Merge1/1 -> Add/1
  2*pi2/1 -> Add/2  "Control Delay  Compensation"
  InertialDqVoltageSource/3(w_u) -> Merge2/2
  [v_abc] -> Bus Creator/1  "v_abc"
  [i_abc] -> Bus Creator/2  "i_abc"
  [w_u] -> Bus Creator/3
  InfiniteDqVoltageSource/3(w_u) -> Merge2/1
  Merge2/1 -> [w_u]  "w_u"
  Bus Creator/1 -> m/1
  Three-Phase V-I Measurement/1 -> [v_abc]
  Three-Phase V-I Measurement/2 -> [i_abc]
  [P] -> Bus Creator/4  "P"
  [Q] -> Bus Creator/5  "Q"
  Divide/1 -> dq02abc_norm/1  "vdq_u_ref"
  dE (pu)/1 -> Sum/1
  Sum/1 -> Divide/1
  Constant/1 -> Sum/2
  Add/1 -> Math Function/1  "Theta"
  Constant2/1 -> Math Function/2
  connections:
  Source_For_LF/RConn2 -- Three-Phase V-I Measurement/LConn2 -- Source_For_OP/RConn2
  Source_For_OP/LConn1 -- Ground/LConn1 -- Source_For_LF/LConn1
  Source_For_LF/RConn3 -- Three-Phase V-I Measurement/LConn3 -- Source_For_OP/RConn3
  Source_For_OP/RConn1 -- Source_For_LF/RConn1 -- Load Flow Bus/LConn1 -- Three-Phase V-I Measurement/LConn1
  Three-Phase V-I Measurement/RConn1 -- A/RConn1
  Three-Phase V-I Measurement/RConn2 -- B/RConn1
  Three-Phase V-I Measurement/RConn3 -- C/RConn1

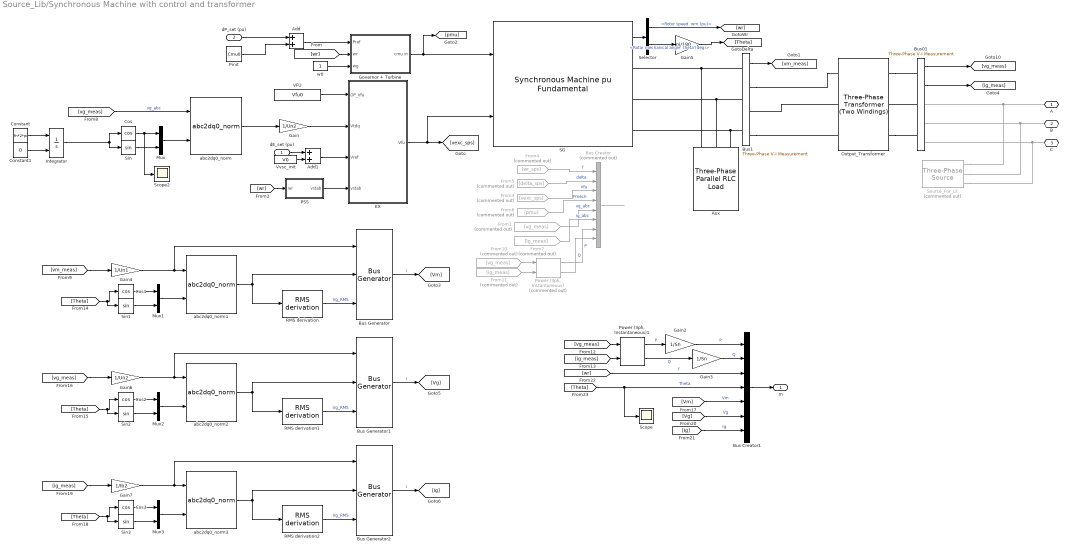
== system Source_Lib/Synchronous Machine with control and transformer ==
  dE_set (pu) : Inport
  dP_set (pu) : Inport  Port=2
  Add : Sum
  Add1 : Sum
  Aux : powerlib/Elements/Three-Phase Parallel RLC Load  LConnTagsString=A|B|C  Configuration=Y (grounded)  NominalVoltage=Un1  Vabc=[1e3 1e3 1e3]  Vabcp=[1e3 1e3 1e3]  NominalFrequency=fn  UnbalancedPower=off  ActivePower=Paux*Sn  InductivePower=0  CapacitivePower=0  Pabc=[10e3 9e3 11e3]  QLabc=[100 90 110]  QCabc=[100 90 110]  Pabcp=[10e3 9e3 11e3]  QLabcp=[100 90 110]  QCabcp=[100 90 110]  Measurements=None  LoadType=constant Z
  Bus Creator : BusCreator  Commented=on  Inputs=8
  Bus Creator1 : BusCreator  Inputs=7
  Bus Generator : Control_Lib/Bus Generator  Gpu=Un1
      settings: SourceProductName=VSC4SPS
  Bus Generator1 : Control_Lib/Bus Generator  Gpu=Un2
      settings: SourceProductName=VSC4SPS
  Bus Generator2 : Control_Lib/Bus Generator  Gpu=Ib2
      settings: SourceProductName=VSC4SPS
  Bus01 : powerlib/Measurements/Three-Phase V-I Measurement  VoltageMeasurement=phase-to-ground  SetLabelV=off  LabelV=Vabc  Vpu=off  VpuLL=off  CurrentMeasurement=yes  SetLabelI=off  LabelI=Iabc  Ipu=off  Pbase=100e6  Vbase=500e3  OutputType=Complex  PhasorSimulation=off  PSBequivalent=0
  Bus1 : powerlib/Measurements/Three-Phase V-I Measurement  VoltageMeasurement=phase-to-ground  SetLabelV=off  LabelV=Vabc  Vpu=off  VpuLL=off  CurrentMeasurement=no  SetLabelI=off  LabelI=Iabc  Ipu=off  Pbase=100e6  Vbase=500e3  OutputType=Complex  PhasorSimulation=off  PSBequivalent=0
  Constant : Constant  Value=fn*2*pi
  Constant1 : Constant  Value=0
  Cos{,1..3} (4 alike) : Trigonometry  Operator=cos
  EX : Subsystem
      mask Display: disp('Excitation system \n ST1C')
  From1 : From  Commented=on  GotoTag=vg_meas
  From10 : From  Commented=on  GotoTag=vg_meas
  From11 : From  Commented=on  GotoTag=ig_meas
  From3 : From  Commented=on  GotoTag=vexc_sps
  From4 : From  Commented=on  GotoTag=wr_sps
  From5 : From  Commented=on  GotoTag=delta_sps
  From6 : From  Commented=on  GotoTag=pmu
  From7 : From  Commented=on  GotoTag=ig_meas
  Gain : Gain  Gain=1/Un2
  Gain2 : Gain  Gain=1/Sn
  Gain3 : Gain  Gain=1/Sn
  Gain4 : Gain  Gain=1/Un1
  Gain5 : Gain  Gain=pi/180
  Gain6 : Gain  Gain=1/Un2
  Gain7 : Gain  Gain=1/Ib2
  Governor + Turbine : Subsystem
      mask Display: disp('IEESGO')
  Integrator : Integrator  InitialConditionSource=external
  Mux{,1..3} (4 alike) : Mux  Inputs=2
  Output_Transformer : powerlib/Elements/Three-Phase Transformer (Two Windings)  Winding1Connection=Yg  Winding2Connection=Yg  CoreType=Three single-phase transformers  SetSaturation=off  Hysteresis=off  DataFile='hysteresis'  SetInitialFlux=off  Measurements=None  UNITS=pu  NominalPower=[Sn , fb]  Winding1=[Un1 , Rt_pu/2 , Lt_pu/2]  Winding2=[Un2 , Rt_pu/2 , Lt_pu/2]  Rm=Rm_pu  Lm=Lm_pu  L0=0.5  Saturation=[ 0,0 ; 0.0024,1.2 ; 1.0,1.52 ]  InitialFluxes=[ 0.8 , -0.8 , 0.7 ]  BreakLoop=off  DiscreteSolver=Trapezoidal iterative  DataType=off  TransfoNumber=1
  PSS : Subsystem
      mask Display: disp('PSS')
  Pinit : Constant  Value=Cmu0
  "Power (3ph, Instantaneous)" : spsPower3phInstantaneousLib/Power (3ph, Instantaneous)  Commented=on
  "Power (3ph, Instantaneous)1" : spsPower3phInstantaneousLib/Power (3ph, Instantaneous)
  RMS derivation : Control_Lib/RMS derivation  SystemSampleTime=-1  VariantActivationTime=update diagram  Latency=0  AutoFrameSizeCalculation=off
      settings: SourceProductName=VSC4SPS
  RMS derivation1 : Control_Lib/RMS derivation  SystemSampleTime=-1  VariantActivationTime=update diagram  Latency=0  AutoFrameSizeCalculation=off
      settings: SourceProductName=VSC4SPS
  RMS derivation2 : Control_Lib/RMS derivation  SystemSampleTime=-1  VariantActivationTime=update diagram  Latency=0  AutoFrameSizeCalculation=off
      settings: SourceProductName=VSC4SPS
  SG : spsSynchronousMachinepuFundamentalLib/Synchronous Machine pu Fundamental  PresetModel=No  MechanicalLoad=Mechanical power Pm  ShowDetailedParameters=on  RotorType=Round  Units=per unit fundamental parameters  MeasurementBus=off  NominalParameters="[Sn  SM_Unom   fn]"  Stator="[ SM_Rs  SM_Ll  SM_Lmd  SM_Lmq]"  Field="[ SM_Rf  SM_Llfd ]"  Dampers2="[ SM_Rkd  SM_Llkd  SM_Rkq1  SM_Llkq1  SM_Rkq2  SM_Llkq2 ]"  Dampers1="[ 1.17E-02  0.182  1.97E-02  0.384 ]"  Mechanical="[SM_H  SM_F  SM_p]"  PolePairs=20  InitialConditions="[0 delta0  ia0  ib0 ic0 pha0 phb0 phc0 Vfu0]"  SetSaturation=off  Saturation=[0.6404,0.7127,0.8441,0.9214,0.9956,1.082,1.19,1.316,1.457;0.7,0.7698,0.8872,0.9466,0.9969,1.046,1.1,1.151,1.201]  LoadFlowParameters=[1,0,0,0,0]  TsPowergui=0  TsBlock=-1  IterativeModel=Trapezoidal non iterative  IterativeDiscreteModel=Trapezoidal non iterative  BusType=PQ  Pref=P0*Sn  Qref=Q0*Sn  Qmin=-Inf  Qmax=Inf  PLF=0  QLF=0
      settings: SourceProductBaseCode=PS
  Scope : Scope
  Scope2 : Scope
  Selector : BusSelector  OutputSignals="Mechanical.Rotor speed  wm (pu),Mechanical.Rotor mechanical angle  theta (deg)"
  Sin{,1..3} (4 alike) : Trigonometry
  Source_For_LF : powerlib/Electrical Sources/Three-Phase Source  Commented=on  InternalConnection=Yg  VoltagePhases=off  Voltage=(400000)*1  PhaseAngle=3.6743  Voltage_phases=[25e3 25e3 25e3]/sqrt(3)  PhaseAngles_phases=[0 -120 +120]  Frequency=fb  NonIdealSource=off  SpecifyImpedance=off  Resistance=0  Inductance=0  ShortCircuitLevel=100e6  BaseVoltage=Un  XRratio=7  BusType=PV  Pref=P0*Sn  Qref=Q0*Sn  Prefabc=[10e3, 10e3, 10e3]  Qrefabc=[0, 0, 0]  Qmin=-inf  Qmax=inf
  VFU : Constant  Value=Vfu0
  Vvsc_init : Constant  Value=V0
  abc2dq0_norm{,1..3} (4 alike) : Control_Lib/abc2dq0_norm  referenceAxisMode=Reference axis at 90 degrees behind phase_a  baseUpdateGain=1
      settings: SourceProductName=VSC4SPS
  w0 : Constant
  A : PMIOPort  Side=Right
  B : PMIOPort  Port=2  Side=Right
  C : PMIOPort  Port=3  Side=Right
  m : Outport
  wires:
  "Power (3ph, Instantaneous)"/2 -> Bus Creator/8  "Q"
  "Power (3ph, Instantaneous)"/1 -> Bus Creator/7  "P"
  From11/1 -> "Power (3ph, Instantaneous)"/2
  From10/1 -> "Power (3ph, Instantaneous)"/1
  [wr] -> PSS/1(wr)
  SG/1 -> Selector/1
  VFU/1 -> EX/1(OP_Vfu)
  [wr] -> Governor + Turbine/2(wr)
  w0/1 -> Governor + Turbine/3(wg)
  Add1/1 -> EX/3(Vref)
  PSS/1(vstab) -> EX/4(vstab)
  Selector/2 -> Gain5/1  "<Rotor mechanical angle  theta (deg)>"
  From4/1 -> Bus Creator/1  "f"
  From5/1 -> Bus Creator/2  "delta"
  From3/1 -> Bus Creator/3  "Vfu"
  From6/1 -> Bus Creator/4  "Pmech"
  Bus Creator/1 -> ?
  Selector/1 -> [wr]  "<Rotor speed  wm (pu)>"
  Bus01/2 -> [ig_meas]
  Bus01/1 -> [vg_meas]
  From1/1 -> Bus Creator/5  "vg_abc"
  From7/1 -> Bus Creator/6  "ig_abc"
  dE_set (pu)/1 -> Add1/1
  Vvsc_init/1 -> Add1/2
  dP_set (pu)/1 -> Add/1
  Pinit/1 -> Add/2
  Add/1 -> Governor + Turbine/1(Pref)
  Constant/1 -> Integrator/1
  Constant1/1 -> Integrator/2
  Cos/1 -> Scope2/1, Mux/1
  Sin/1 -> Mux/2
  Mux/1 -> abc2dq0_norm/2
  Integrator/1 -> Sin/1, Cos/1
  [vg_meas] -> abc2dq0_norm/1  "vg_abc"
  Gain/1 -> EX/2(Vtdq)
  abc2dq0_norm/2 -> Gain/1
  Governor + Turbine/1(cmu in) -> SG/1, [pmu]
  EX/1(Vfu) -> SG/2, [vexc_sps]
  Bus1/1 -> [vm_meas]
  Bus Generator2/1 -> [Ig]  "I"
  RMS derivation2/1 -> Bus Generator2/3  "Vg_RMS"
  abc2dq0_norm3/2 -> Bus Generator2/2, RMS derivation2/1
  [Theta] -> Cos3/1, Sin3/1
  Cos3/1 -> Mux3/1
  Sin3/1 -> Mux3/2
  Mux3/1 -> abc2dq0_norm3/2
  Gain7/1 -> abc2dq0_norm3/1, Bus Generator2/1
  [ig_meas] -> Gain7/1
  [vg_meas] -> Gain6/1
  Gain6/1 -> Bus Generator1/1, abc2dq0_norm2/1
  Mux2/1 -> abc2dq0_norm2/2
  Sin2/1 -> Mux2/2
  Cos2/1 -> Mux2/1
  [Theta] -> Sin2/1, Cos2/1
  abc2dq0_norm2/2 -> RMS derivation1/1, Bus Generator1/2
  RMS derivation1/1 -> Bus Generator1/3  "Vg_RMS"
  Bus Generator1/1 -> [Vg]  "I"
  Bus Generator/1 -> [Vm]  "I"
  RMS derivation/1 -> Bus Generator/3  "Vg_RMS"
  abc2dq0_norm1/2 -> Bus Generator/2, RMS derivation/1
  [Theta] -> Cos1/1, Sin1/1
  Cos1/1 -> Mux1/1
  Sin1/1 -> Mux1/2
  Mux1/1 -> abc2dq0_norm1/2
  Gain4/1 -> abc2dq0_norm1/1, Bus Generator/1
  [vm_meas] -> Gain4/1
  [Ig] -> Bus Creator1/7  "Ig"
  [Vg] -> Bus Creator1/6  "Vg"
  [Vm] -> Bus Creator1/5  "Vm"
  [Theta] -> Scope/1, Bus Creator1/4  "Theta"
  [wr] -> Bus Creator1/3  "f"
  Gain3/1 -> Bus Creator1/2  "Q"
  Gain2/1 -> Bus Creator1/1  "P"
  Bus Creator1/1 -> m/1
  [vg_meas] -> "Power (3ph, Instantaneous)1"/1
  [ig_meas] -> "Power (3ph, Instantaneous)1"/2
  "Power (3ph, Instantaneous)1"/1 -> Gain2/1  "P"
  "Power (3ph, Instantaneous)1"/2 -> Gain3/1  "Q"
  Gain5/1 -> [Theta]
  connections:
  Aux/LConn1 -- Bus1/LConn1 -- SG/RConn1
  Aux/LConn2 -- Bus1/LConn2 -- SG/RConn2
  Aux/LConn3 -- Bus1/LConn3 -- SG/RConn3
  Source_For_LF/RConn1 -- A/RConn1 -- Bus01/RConn1
  Source_For_LF/RConn3 -- C/RConn1 -- Bus01/RConn3
  Source_For_LF/RConn2 -- B/RConn1 -- Bus01/RConn2
  Output_Transformer/RConn1 -- Bus01/LConn1
  Bus01/LConn2 -- Output_Transformer/RConn2
  Output_Transformer/RConn3 -- Bus01/LConn3
  Bus1/RConn1 -- Output_Transformer/LConn1
  Output_Transformer/LConn2 -- Bus1/RConn2
  Bus1/RConn3 -- Output_Transformer/LConn3
